simulink model "null_test"  (R2018b)
settings: Solver=VariableStepAuto  StartTime=0.0  StopTime=10.0  RelTol=1e-3
undefined symbols (not defined in the file or in its folder): fswParams
libraries: rwa_allocation_lib x1
settings Model: Creator=Nick's PC  LastModifiedBy=Nick's PC

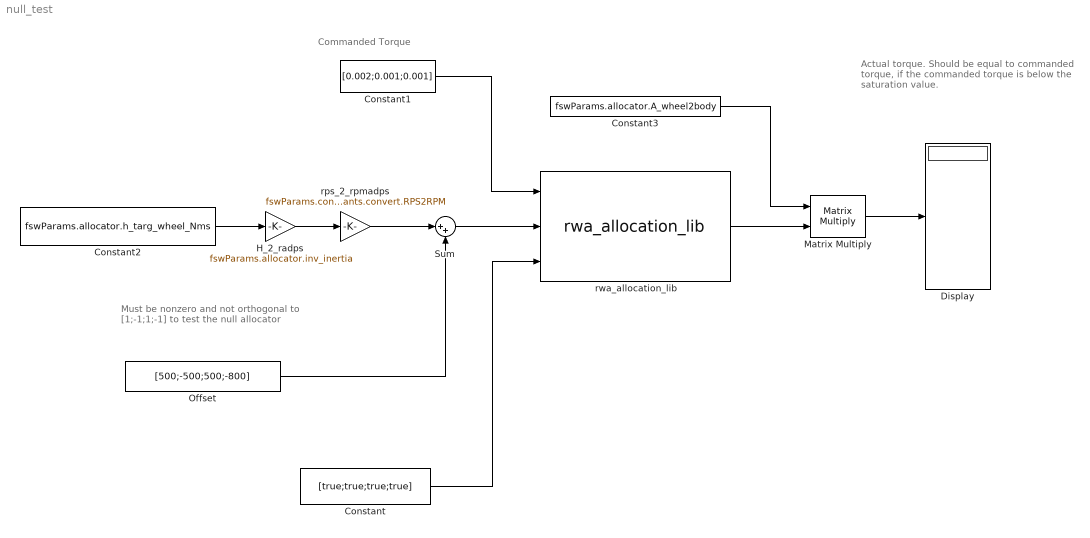
== system null_test ==
  note: Must be nonzero and not orthogonal to [1;-1;1;-1] to test the null allocator
  note: Actual torque. Should be equal to commanded torque, if the commanded torque is below the saturation value.
  note: Commanded Torque
  Constant : Constant  Value=[true;true;true;true]
  Constant1 : Constant  Value=[0.002;0.001;0.001]
  Constant2 : Constant  Value=fswParams.allocator.h_targ_wheel_Nms
  Constant3 : Constant  Value=fswParams.allocator.A_wheel2body
  Display : Display
  H_2_radps : Gain  Gain=fswParams.allocator.inv_inertia
  Matrix Multiply : Product  Multiplication=Matrix(*)
  Offset : Constant  Value=[500;-500;500;-800]
  Sum : Sum  Inputs=|++
  rps_2_rpmadps : Gain  Gain=fswParams.constants.convert.RPS2RPM
  rwa_allocation_lib : rwa_allocation_lib/rwa_allocation_lib  SystemSampleTime=-1
      link override If Action Subsystem/feedback_gain: Gain=0*fswParams.allocator.feedback_gain
  wires:
  Constant/1 -> rwa_allocation_lib/3
  H_2_radps/1 -> rps_2_rpmadps/1
  rps_2_rpmadps/1 -> Sum/1
  Sum/1 -> rwa_allocation_lib/2
  Constant3/1 -> Matrix Multiply/1
  Constant2/1 -> H_2_radps/1
  Constant1/1 -> rwa_allocation_lib/1
  rwa_allocation_lib/1 -> Matrix Multiply/2
  Offset/1 -> Sum/2
  Matrix Multiply/1 -> Display/1
